simulink model "FloatingvsFixed"  (R2020b)
settings: Solver=VariableStepAuto  StartTime=0.0  StopTime=20  RelTol=1e-3
settings Model: Creator=alan  LastModifiedBy=alan

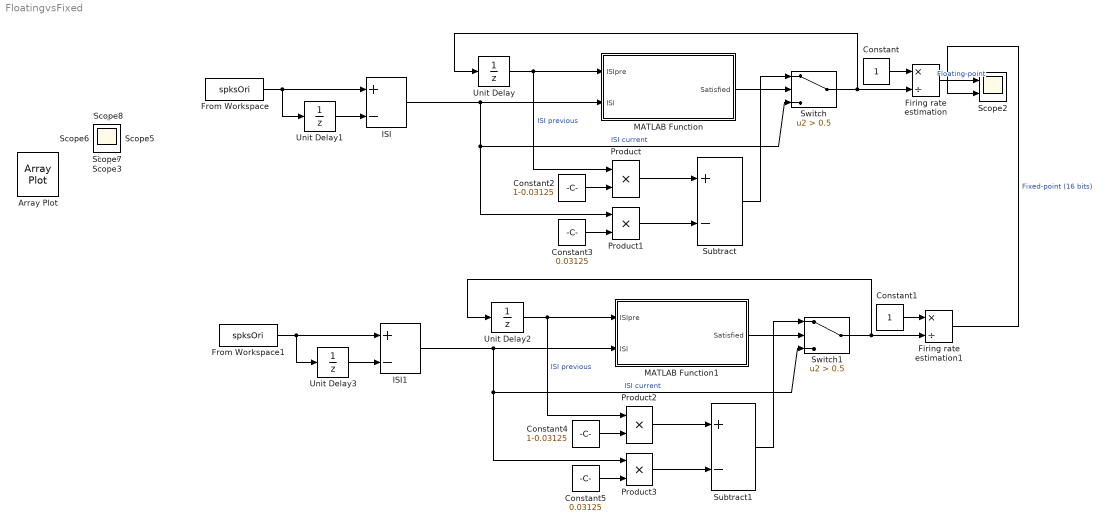
== system FloatingvsFixed ==
  Constant : Constant
  Constant1 : Constant
  Constant2 : Constant  Value=1-0.03125
  Constant3 : Constant  Value=0.03125
  Constant4 : Constant  Value=1-0.03125
  Constant5 : Constant  Value=0.03125
  Firing rate estimation : Product  Inputs=*/
  Firing rate estimation1 : Product  Inputs=*/  OutDataTypeStr=fixdt(0,16,4)
  From Workspace : FromWorkspace  VariableName=spksOri
  From Workspace1 : FromWorkspace  VariableName=spksOri
  ISI : Sum  Inputs=+-  AccumDataTypeStr=double  OutDataTypeStr=double
  ISI1 : Sum  Inputs=+-  AccumDataTypeStr=fixdt(0,16,10)  OutDataTypeStr=fixdt(0,16,15)
  MATLAB Function : MATLAB Function  TreatAsAtomicUnit=on
  MATLAB Function1 : MATLAB Function  TreatAsAtomicUnit=on
  Product{,1..3} (4 alike) : Product  OutDataTypeStr=double
  Scope2 : Scope  NumInputPorts=2
  Subtract : Sum  Inputs=+-
  Subtract1 : Sum  Inputs=+-  OutDataTypeStr=fixdt(0,16,15)
  Switch : Switch  Criteria=u2 > Threshold  Threshold=0.5  RndMeth=Round
  Switch1 : Switch  Criteria=u2 > Threshold  Threshold=0.5  OutDataTypeStr=fixdt(0,16,15)  RndMeth=Round
  Unit Delay{,1..3} (4 alike) : UnitDelay  SampleTime=0.2857  HasFrameUpgradeWarning=on
  Array Plot : ArrayPlot  IOType=viewer
  Scope{,1,3,5..8} (7 alike) : Scope
  wires:
  ISI/1 -> Switch/3, Product1/1, MATLAB Function/2(ISI)  "ISI current"
  Constant3/1 -> Product1/2
  Product/1 -> Subtract/1
  Constant2/1 -> Product/2
  Unit Delay/1 -> Product/1, MATLAB Function/1(ISIpre)  "ISI previous"
  Switch/1 -> Firing rate estimation/2, Unit Delay/1
  From Workspace/1 -> Unit Delay1/1, ISI/1
  Unit Delay1/1 -> ISI/2
  Product1/1 -> Subtract/2
  Subtract/1 -> Switch/1
  MATLAB Function/1(Satisfied) -> Switch/2
  Constant/1 -> Firing rate estimation/1
  Firing rate estimation/1 -> Scope2/1  "Floating-point"
  From Workspace1/1 -> Unit Delay3/1, ISI1/1
  Unit Delay3/1 -> ISI1/2
  Constant5/1 -> Product3/2
  Unit Delay2/1 -> Product2/1, MATLAB Function1/1(ISIpre)  "ISI previous"
  Subtract1/1 -> Switch1/1
  Product2/1 -> Subtract1/1
  Product3/1 -> Subtract1/2
  Constant4/1 -> Product2/2
  MATLAB Function1/1(Satisfied) -> Switch1/2
  Switch1/1 -> Firing rate estimation1/2, Unit Delay2/1
  Constant1/1 -> Firing rate estimation1/1
  ISI1/1 -> Switch1/3, Product3/1, MATLAB Function1/2(ISI)  "ISI current"
  Firing rate estimation1/1 -> Scope2/2  "Fixed-point (16 bits)"

== matlab function FloatingvsFixed/MATLAB Function ==
  data: Satisfied output; ISIpre input; ISI input
function Satisfied = Penalised_Condition( ISIpre, ISI)

if (ISIpre-ISI) >= (ISIpre*ISI*32)
    Satisfied = 1;
else
    Satisfied = 0;
end

== matlab function FloatingvsFixed/MATLAB Function1 ==
  data: Satisfied output; ISIpre input; ISI input
function Satisfied = Penalised_Condition( ISIpre, ISI)

if (ISIpre-ISI) >= (ISIpre*ISI*32)
    Satisfied = 1;
else
    Satisfied = 0;
end
